simulink model "thermo"  (Simulink 6.0)
settings: Solver=ode45  SolverMode=SingleTasking  StartTime=0.0  StopTime=2*24*60*60  FixedStep=100  RelTol=1e-3  AbsTol=1e-6
PreLoadFcn:
  | thermdat
values from neighbouring files (symbols this model uses):
  c = 2    [pndanim2.m]    (also in pndanim3.m = 3; thermdat.m = 1005.4)
  cost = 0.09/3.6e6    (= 2.5e-08)    [thermdat.m]
  ha = THeater*c    (= 304636.2)    [thermdat.m]
  M = (lenHouse*widHouse*htHouse+tan(pitRoof)*widHouse*lenHouse)*densAir    [thermdat.m]
  Mdot = 0.1    [thermdat.m]
  Req = RWall*RWindow/(RWall + RWindow)    [thermdat.m]
  TinIC = 20    [thermdat.m]
libraries: simulink_extras x3
settings Model: Creator=The MathWorks Inc.  LastModifiedBy=batserve  ExtModeTrigMode=oneshot  ExtModeArmWhenConnect=off  ExtModeAutoUpdateStatusClock=off
settings DataIOCC: ExternalInput=[]  InitialState=[]  LimitDataPoints=off  SaveOutput=off  SaveTime=off
settings OptimizationCC: BlockReduction=off  BooleanDataType=off
settings DebuggingCC: CheckExecutionContextPreStartOutputMsg=on  CheckExecutionContextRuntimeOutputMsg=on  SolverPrmCheckMsg=none  IntegerOverflowMsg=none
settings HardwareCC: TargetUnknown=on

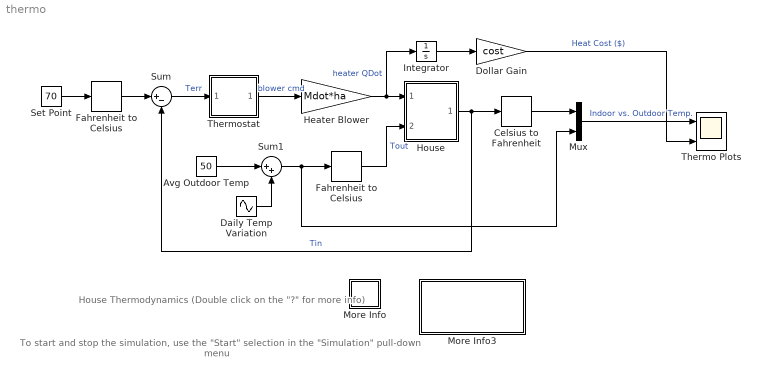
== system thermo ==
  note: House Thermodynamics
      | (Double click on the "?" for more info)
  note: To start and stop the simulation, use the "Start"
      | selection in the "Simulation" pull-down menu
  Avg Outdoor Temp : Constant  Value=50
  Celsius to Fahrenheit : simulink_extras/Transformations/Celsius to Fahrenheit
  Daily Temp Variation : Sin  Amplitude=15  Frequency=2*pi/(24*3600)  SampleTime=0
  Dollar Gain : Gain  Gain=cost  SaturateOnIntegerOverflow=on
  Fahrenheit to Celsius : simulink_extras/Transformations/Fahrenheit to Celsius
  "Fahrenheit to Celsius " : simulink_extras/Transformations/Fahrenheit to Celsius
  Heater Blower : Gain  Gain=Mdot*ha  SaturateOnIntegerOverflow=on
  House : Subsystem  PropExecContextAcrossSSBoundary=on
      mask Display: plot(0,0,100,100,[20,80,80,20,20],[20,20,70,70,20],[15,50,85,15],[70,90,70,70],[42,42,29,29],[20,44,44,20],[52,68,68,52,52],[55,55,44,44,55])
  Integrator : Integrator
  More Info : Subsystem  PropExecContextAcrossSSBoundary=on
      mask Display: disp('?')
  More Info3 : Subsystem  PropExecContextAcrossSSBoundary=on
      settings: OpenFcn=simcad(bdroot);
      mask Display: disp('Double click\nhere for\nSimulink Help')
  Mux : Mux  Inputs=2
  Set Point : Constant  Value=70
  Sum : Sum  Inputs=|+-  SaturateOnIntegerOverflow=on  InputSameDT=on
  Sum1 : Sum  Inputs=|++  SaturateOnIntegerOverflow=on  InputSameDT=on
  Thermo Plots : Scope  NumInputPorts=2
      settings: TickLabels=on  TimeRange=172800  YMin=20~0  YMax=80~30  DataFormat=Array
  Thermostat : Subsystem  PropExecContextAcrossSSBoundary=on
      mask Display: plot(0,0,100,100,[20,80,80,20,20],[20,20,80,80,20],[70,65,50,35,30],[20,40,50,40,20],[45,40,43],[47,59,45],[30,30],[60,60],[40,40],[65,65],[50,50],[70,70],[60,60],[65,65],[70,70],[60,60])
  wires:
  Set Point/1 -> "Fahrenheit to Celsius "/1
  "Fahrenheit to Celsius "/1 -> Sum/1
  Integrator/1 -> Dollar Gain/1
  Heater Blower/1 -> Integrator/1, House/1(Heater QDot In)  "heater QDot"
  Thermostat/1(Blower switch) -> Heater Blower/1  "blower cmd"
  Sum/1 -> Thermostat/1(Terr)  "Terr"
  House/1(Indoor Temp Tin) -> Sum/2, Celsius to Fahrenheit/1  "Tin"
  Daily Temp Variation/1 -> Sum1/2
  Sum1/1 -> Fahrenheit to Celsius/1, Mux/2
  Avg Outdoor Temp/1 -> Sum1/1
  Celsius to Fahrenheit/1 -> Mux/1
  Fahrenheit to Celsius/1 -> House/2(Outdoor Temp Tout)  "Tout"
  Mux/1 -> Thermo Plots/1  "Indoor vs. Outdoor Temp."
  Dollar Gain/1 -> Thermo Plots/2  "Heat Cost ($)"

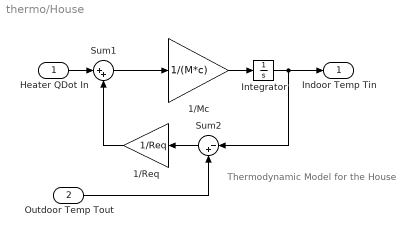
== system thermo/House ==
  note: Thermodynamic Model
      | for the House
  Heater QDot In : Inport  Port=1  LatchInput=off
  Outdoor Temp Tout : Inport  Port=2  LatchInput=off
  1/Mc : Gain  Gain=1/(M*c)  SaturateOnIntegerOverflow=on
  1/Req : Gain  Orientation=left  Gain=1/Req  SaturateOnIntegerOverflow=on
  Integrator : Integrator  InitialCondition=TinIC
  Sum1 : Sum  Inputs=|++  SaturateOnIntegerOverflow=on  InputSameDT=on
  Sum2 : Sum  Orientation=left  Inputs=|-+  SaturateOnIntegerOverflow=on  InputSameDT=on
  Indoor Temp Tin : Outport  InitialOutput=0
  wires:
  Outdoor Temp Tout/1 -> Sum2/2
  Heater QDot In/1 -> Sum1/1
  Sum1/1 -> 1/Mc/1
  Sum2/1 -> 1/Req/1
  1/Req/1 -> Sum1/2
  1/Mc/1 -> Integrator/1
  Integrator/1 -> Sum2/1, Indoor Temp Tin/1

== system thermo/More Info ==
  note: This system models the thermodynamics of a house.
      | The variables are initialized by a file
      | called thermdat.m.
  note: Examine the file thermdat.m to see the
      | simulation variables you can change at will.

== system thermo/More Info3 ==

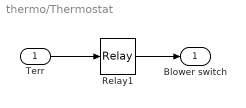
== system thermo/Thermostat ==
  Terr : Inport  Port=1  LatchInput=off
  Relay1 : Relay  OnSwitchValue=5*(5/9)  OffSwitchValue=-5*(5/9)
  Blower switch : Outport  InitialOutput=0
  wires:
  Terr/1 -> Relay1/1
  Relay1/1 -> Blower switch/1
